simulink model "modele_simplifie"  (R2025b)
settings: Solver=VariableStepAuto  StartTime=0.0  StopTime=T_att  RelTol=1e-3
values from neighbouring files (symbols this model uses):
  d = 4    [script_devoir2.m]
  g = 9.81    [script_devoir2.m]
  isQ3a = false    [script_devoir2.m]
  Kdx = -0.367    [script_devoir2.m]
  Kdy = 15000    [script_devoir2.m]
  Kix = -0.176    [script_devoir2.m]
  Kiy = 125000    [script_devoir2.m]
  Kpx = -0.440    (= -0.44)    [script_devoir2.m]
  Kpy = 75000    [script_devoir2.m]
  m = 1000    [script_devoir2.m]
  T_att = 20    [script_devoir2.m]
  x0 = [x0_pos; vx0; y0_pos; vy0; 0; 0]    [script_devoir2.m]
  x0_pos = 10    [script_devoir2.m]
  y0_pos = 50    [script_devoir2.m]
settings Model: Creator=andreagourion  LastModifiedBy=diegoalfonsocosta

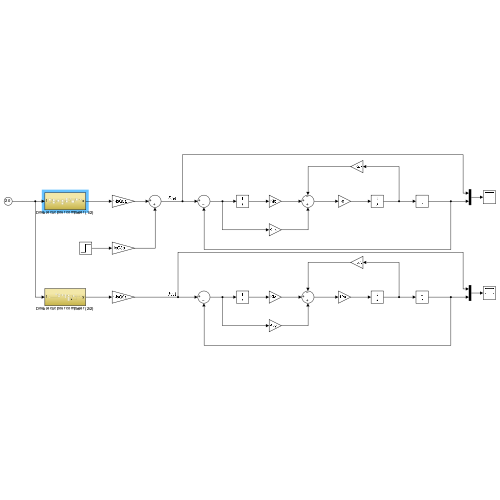
[thumbnail: Simulink's stored preview of the top-level diagram]
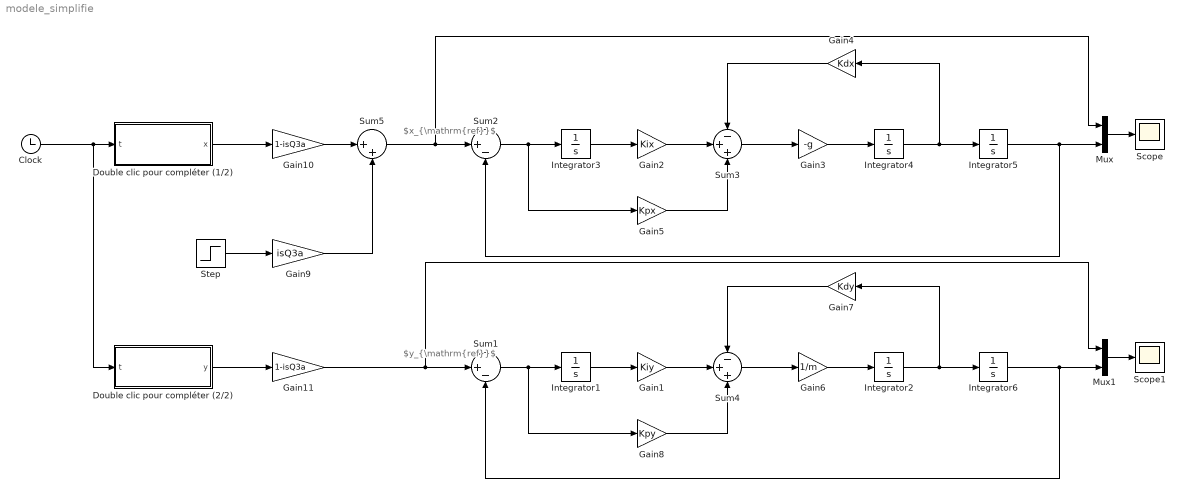
== system modele_simplifie ==
  note: $x_{\mathrm{ref}}$
  note: $y_{\mathrm{ref}}$
  Clock : Clock
  Double clic pour compléter (1/2) : Subsystem
  Double clic pour compléter (2/2) : Subsystem
  Gain1 : Gain  Gain=Kiy
  Gain10 : Gain  Gain=1-isQ3a
  Gain11 : Gain  Gain=1-isQ3a
  Gain2 : Gain  Gain=Kix
  Gain3 : Gain  Gain=-g
  Gain4 : Gain  Gain=Kdx
  Gain5 : Gain  Gain=Kpx
  Gain6 : Gain  Gain=1/m
  Gain7 : Gain  Gain=Kdy
  Gain8 : Gain  Gain=Kpy
  Gain9 : Gain  Gain=isQ3a
  Integrator1 : Integrator
  Integrator2 : Integrator  InitialCondition=x0(4)
  Integrator3 : Integrator
  Integrator4 : Integrator  InitialCondition=x0(2)
  Integrator5 : Integrator  InitialCondition=x0(1)
  Integrator6 : Integrator  InitialCondition=x0(3)
  Mux : Mux  Inputs=2
  Mux1 : Mux  Inputs=2
  Scope : Scope
      settings: SampleTime=Ts  ActiveDisplayYMinimum=-1  ActiveDisplayYMaximum=1  DataLoggingVariableName=xsimp  DataLoggingSaveFormat=Array
  Scope1 : Scope
      settings: SampleTime=Ts  ActiveDisplayYMinimum=-1  ActiveDisplayYMaximum=1  DataLoggingVariableName=ysimp  DataLoggingSaveFormat=Array
  Step : Step  Time=0  SampleTime=0
  Sum1 : Sum  Inputs=|+-
  Sum2 : Sum  Inputs=|+-
  Sum3 : Sum  Inputs=-++
  Sum4 : Sum  Inputs=-++
  Sum5 : Sum  Inputs=|++
  wires:
  Clock/1 -> Double clic pour compléter (1/2)/1(t), Double clic pour compléter (2/2)/1(t)
  Integrator3/1 -> Gain2/1
  Sum2/1 -> Gain5/1, Integrator3/1
  Integrator4/1 -> Gain4/1, Integrator5/1
  Gain2/1 -> Sum3/2
  Sum3/1 -> Gain3/1
  Gain3/1 -> Integrator4/1
  Gain4/1 -> Sum3/1
  Gain5/1 -> Sum3/3
  Integrator5/1 -> Mux/2, Sum2/2
  Sum1/1 -> Gain8/1, Integrator1/1
  Sum4/1 -> Gain6/1
  Integrator1/1 -> Gain1/1
  Gain6/1 -> Integrator2/1
  Integrator2/1 -> Gain7/1, Integrator6/1
  Gain1/1 -> Sum4/2
  Gain7/1 -> Sum4/1
  Gain8/1 -> Sum4/3
  Mux/1 -> Scope/1
  Mux1/1 -> Scope1/1
  Integrator6/1 -> Sum1/2, Mux1/2
  Double clic pour compléter (2/2)/1(y) -> Gain11/1
  Step/1 -> Gain9/1
  Double clic pour compléter (1/2)/1(x) -> Gain10/1
  Sum5/1 -> Mux/1, Sum2/1
  Gain9/1 -> Sum5/2
  Gain10/1 -> Sum5/1
  Gain11/1 -> Mux1/1, Sum1/1

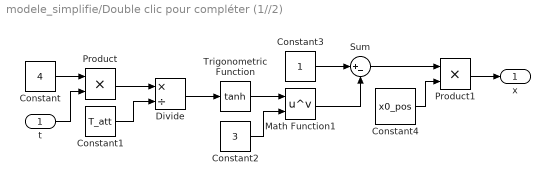
== system modele_simplifie/Double clic pour compléter (1//2) ==
  t : Inport
  Constant : Constant  Value=4
  Constant1 : Constant  Value=T_att
  Constant2 : Constant  Value=3
  Constant3 : Constant
  Constant4 : Constant  Value=x0_pos
  Divide : Product  Inputs=*/
  Math Function1 : Math  Operator=pow
  Product : Product
  Product1 : Product
  Sum : Sum  Inputs=|+-
  Trigonometric Function : Trigonometry  Operator=tanh
  x : Outport
  wires:
  Product/1 -> Divide/1
  t/1 -> Product/2
  Constant/1 -> Product/1
  Constant1/1 -> Divide/2
  Divide/1 -> Trigonometric Function/1
  Trigonometric Function/1 -> Math Function1/1
  Constant2/1 -> Math Function1/2
  Constant3/1 -> Sum/1
  Math Function1/1 -> Sum/2
  Sum/1 -> Product1/1
  Constant4/1 -> Product1/2
  Product1/1 -> x/1

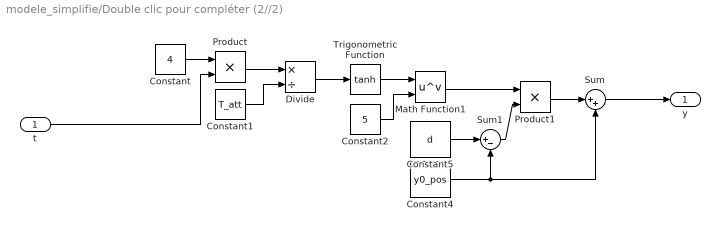
== system modele_simplifie/Double clic pour compléter (2//2) ==
  t : Inport
  Constant : Constant  Value=4
  Constant1 : Constant  Value=T_att
  Constant2 : Constant  Value=5
  Constant4 : Constant  Value=y0_pos
  Constant5 : Constant  Value=d
  Divide : Product  Inputs=*/
  Math Function1 : Math  Operator=pow
  Product : Product
  Product1 : Product
  Sum : Sum  Inputs=|++
  Sum1 : Sum  Inputs=|+-
  Trigonometric Function : Trigonometry  Operator=tanh
  y : Outport
  wires:
  Trigonometric Function/1 -> Math Function1/1
  Constant2/1 -> Math Function1/2
  Divide/1 -> Trigonometric Function/1
  Product1/1 -> Sum/1
  Product/1 -> Divide/1
  t/1 -> Product/2
  Constant/1 -> Product/1
  Constant1/1 -> Divide/2
  Math Function1/1 -> Product1/1
  Constant4/1 -> Sum/2, Sum1/2
  Constant5/1 -> Sum1/1
  Sum1/1 -> Product1/2
  Sum/1 -> y/1
